simulink model "convdoc"  (Simulink 5.0)
settings: Solver=ode45  SolverMode=SingleTasking  StartTime=0.0  StopTime=inf  RelTol=1e-3
undefined symbols (not defined in the file or in its folder): slcm
libraries: commcnvcod2 x2, commchan2 x1, commdigbbndpm2 x1, commrandsrc2 x1, commsink2 x1
settings Model: Creator=ptrow  LastModifiedBy=ptrow  SaveTime=off  SaveOutput=off  AlgebraicLoopMsg=error  RTWInlineParameters=on  BooleanDataType=off  RTWOptions=-aRollThreshold=5

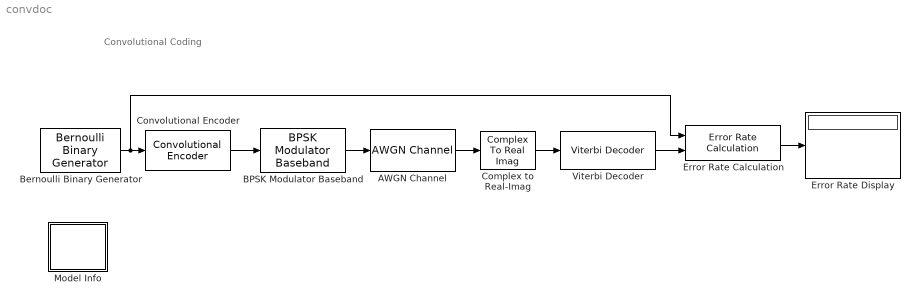
== system convdoc ==
  note: Convolutional Coding
  AWGN Channel : commchan2/AWGN Channel  seed=113  noiseMode="Signal to noise ratio  (Es/No)"  EsNodB=-1  SNRdB=10  Ps=1  Tsym=0.5  variance=1
  BPSK Modulator Baseband : commdigbbndpm2/BPSK Modulator Baseband  Ph=0  numSamp=1
  Bernoulli Binary Generator : commrandsrc2/Bernoulli Binary Generator  P=0.5  seed=61  Ts=1  frameBased=on  sampPerFrame=1  orient=off
  Complex to Real-Imag : ComplexToRealImag  Output=Real
  Convolutional Encoder : commcnvcod2/Convolutional Encoder  trellis=poly2trellis(7, [171 133])  reset=None
  Error Rate Calculation : commsink2/Error Rate Calculation  N=96  st_delay=0  cp_mode=Entire frame  subframe=[]  PMode=Port  WsName=ErrorVec  RsMode2=off  stop=on  numErr=100  maxBits=1e5
  Error Rate Display : Display
  Model Info : Subsystem  LoadFcn=slcm LoadBlock;  InitFcn=slcm('UpdateAllCMBlocksInThisModelInit')  mask(CMBlock){InitialSaveTempField=, InitialBlockCM=None, BlockCM=None, Frame=on, SaveTempField=, DisplayStringWithTags=Info, MaskDisplayString=Info, HorizontalTextAlignment=Center, LeftAlignmentValue=0.5, SourceBlockDiagram=convdoc, TagMaxNumber=20, CMTag1=, CMTag2=, CMTag3=, CMTag4=, CMTag5=, CMTag6=, CMTag7=, CMTag8=, CMTag9=, CMTag10=, CMTag11=, CMTag12=, CMTag13=, CMTag14=, CMTag15=, CMTag16=, CMTag17=, CMTag18=, CMTag19=, CMTag20=}
      mask help: This block allows revision control information to be displayed within the model.
      settings: CopyFcn=slcm CopyBlock;  DeleteFcn=slcm Cancel;  PostSaveFcn=slcm('UpdateAllCMBlocksInThisModel')  NameChangeFcn=slcm Rename;  OpenFcn=commdemohelp;
      mask Display: text(str2num(LeftAlignmentValue), 0.5, MaskDisplayString, 'HorizontalAlignment', HorizontalTextAlignment)
  Viterbi Decoder : commcnvcod2/Viterbi Decoder  trellis=poly2trellis(7, [171 133])  dectype=Unquantized  nsdecb=4  tbdepth=96  opmode=Continuous  reset=off
  wires:
  Bernoulli Binary Generator/1 -> Convolutional Encoder/1, Error Rate Calculation/1
  Convolutional Encoder/1 -> BPSK Modulator Baseband/1
  AWGN Channel/1 -> Complex to Real-Imag/1
  BPSK Modulator Baseband/1 -> AWGN Channel/1
  Error Rate Calculation/1 -> Error Rate Display/1
  Viterbi Decoder/1 -> Error Rate Calculation/2
  Complex to Real-Imag/1 -> Viterbi Decoder/1

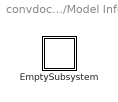
== system convdoc/Model Info ==
  EmptySubsystem : Subsystem

== system convdoc/Model Info/EmptySubsystem ==
